simulink model "quad2_jump"  (R2015b)
settings: Solver=FixedStepAuto  StartTime=0.0  StopTime=10  FixedStep=1e-4  MinStep=1e-4  RelTol=1e-2  AbsTol=1e-6
InitFcn:
  | init_quad;
StartFcn:
  | init_quad;
undefined symbols (not defined in the file or in its folder): body, ctrl, planner, sigbuilder_block, X, Y, Z
libraries: nesl_utility x61, sm_lib x41, simulink x4, Contact_Forces_Lib x4, Parts_Lib x4
(part 3 of 3)

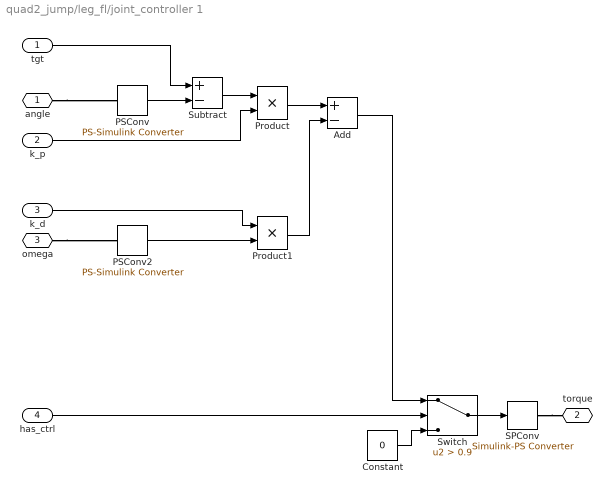
== system quad2_jump/leg_fl/joint_controller 1 ==
  tgt : Inport
  k_p : Inport  Port=2
  k_d : Inport  Port=3
  has_ctrl : Inport  Port=4
  Add : Sum  Inputs=+-
  Constant : Constant  Value=0
  PSConv : nesl_utility/PS-Simulink Converter  PhysicalDomain=network_engine_domain  SubClassName=ps_output  LeftPortType=input  RightPortType=output  PseudoPeriodic=off  Frequencies=[]  Unit=1  AffineConversion=off
  PSConv2 : nesl_utility/PS-Simulink Converter  PhysicalDomain=network_engine_domain  SubClassName=ps_output  LeftPortType=input  RightPortType=output  PseudoPeriodic=off  Frequencies=[]  Unit=1  AffineConversion=off
  Product : Product  Inputs=**
  Product1 : Product  Inputs=**
  SPConv : nesl_utility/Simulink-PS Converter  PhysicalDomain=network_engine_domain  SubClassName=ps_input  LeftPortType=input  RightPortType=output  PseudoPeriodic=off  Frequencies=[]  NoiseDistribution=none  NoiseParameters=[]  Unit=1  AffineConversion=off  InputFiltering=on  SimscapeFilterOrder=2  InputFilterTimeConstant=0.001  UdotUserProvided=1
  Subtract : Sum  Inputs=+-
  Switch : Switch  Criteria=u2 > Threshold  Threshold=0.9
  angle : PMIOPort  Port=1  Side=Left
  torque : PMIOPort  Port=2  Side=Right
  omega : PMIOPort  Port=3  Side=Left
  wires:
  Product1/1 -> Add/2
  tgt/1 -> Subtract/1
  Product/1 -> Add/1
  PSConv/1 -> Subtract/2
  Subtract/1 -> Product/1
  k_d/1 -> Product1/1
  PSConv2/1 -> Product1/2
  k_p/1 -> Product/2
  Switch/1 -> SPConv/1
  has_ctrl/1 -> Switch/2
  Constant/1 -> Switch/3
  Add/1 -> Switch/1
  connections:
  angle/RConn1 -- PSConv/LConn1
  omega/RConn1 -- PSConv2/LConn1
  SPConv/RConn1 -- torque/RConn1

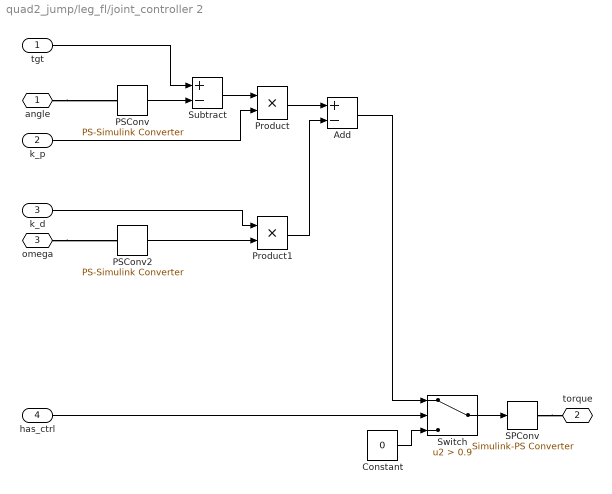
== system quad2_jump/leg_fl/joint_controller 2 ==
  tgt : Inport
  k_p : Inport  Port=2
  k_d : Inport  Port=3
  has_ctrl : Inport  Port=4
  Add : Sum  Inputs=+-
  Constant : Constant  Value=0
  PSConv : nesl_utility/PS-Simulink Converter  PhysicalDomain=network_engine_domain  SubClassName=ps_output  LeftPortType=input  RightPortType=output  PseudoPeriodic=off  Frequencies=[]  Unit=1  AffineConversion=off
  PSConv2 : nesl_utility/PS-Simulink Converter  PhysicalDomain=network_engine_domain  SubClassName=ps_output  LeftPortType=input  RightPortType=output  PseudoPeriodic=off  Frequencies=[]  Unit=1  AffineConversion=off
  Product : Product  Inputs=**
  Product1 : Product  Inputs=**
  SPConv : nesl_utility/Simulink-PS Converter  PhysicalDomain=network_engine_domain  SubClassName=ps_input  LeftPortType=input  RightPortType=output  PseudoPeriodic=off  Frequencies=[]  NoiseDistribution=none  NoiseParameters=[]  Unit=1  AffineConversion=off  InputFiltering=on  SimscapeFilterOrder=2  InputFilterTimeConstant=0.001  UdotUserProvided=1
  Subtract : Sum  Inputs=+-
  Switch : Switch  Criteria=u2 > Threshold  Threshold=0.9
  angle : PMIOPort  Port=1  Side=Left
  torque : PMIOPort  Port=2  Side=Right
  omega : PMIOPort  Port=3  Side=Left
  wires:
  Product1/1 -> Add/2
  tgt/1 -> Subtract/1
  Product/1 -> Add/1
  PSConv/1 -> Subtract/2
  Subtract/1 -> Product/1
  k_d/1 -> Product1/1
  PSConv2/1 -> Product1/2
  k_p/1 -> Product/2
  Switch/1 -> SPConv/1
  has_ctrl/1 -> Switch/2
  Constant/1 -> Switch/3
  Add/1 -> Switch/1
  connections:
  angle/RConn1 -- PSConv/LConn1
  omega/RConn1 -- PSConv2/LConn1
  SPConv/RConn1 -- torque/RConn1

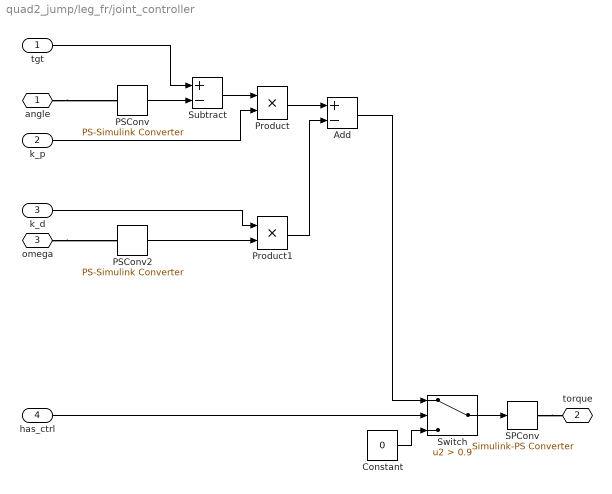
== system quad2_jump/leg_fr/joint_controller  ==
  tgt : Inport
  k_p : Inport  Port=2
  k_d : Inport  Port=3
  has_ctrl : Inport  Port=4
  Add : Sum  Inputs=+-
  Constant : Constant  Value=0
  PSConv : nesl_utility/PS-Simulink Converter  PhysicalDomain=network_engine_domain  SubClassName=ps_output  LeftPortType=input  RightPortType=output  PseudoPeriodic=off  Frequencies=[]  Unit=1  AffineConversion=off
  PSConv2 : nesl_utility/PS-Simulink Converter  PhysicalDomain=network_engine_domain  SubClassName=ps_output  LeftPortType=input  RightPortType=output  PseudoPeriodic=off  Frequencies=[]  Unit=1  AffineConversion=off
  Product : Product  Inputs=**
  Product1 : Product  Inputs=**
  SPConv : nesl_utility/Simulink-PS Converter  PhysicalDomain=network_engine_domain  SubClassName=ps_input  LeftPortType=input  RightPortType=output  PseudoPeriodic=off  Frequencies=[]  NoiseDistribution=none  NoiseParameters=[]  Unit=1  AffineConversion=off  InputFiltering=on  SimscapeFilterOrder=2  InputFilterTimeConstant=0.001  UdotUserProvided=1
  Subtract : Sum  Inputs=+-
  Switch : Switch  Criteria=u2 > Threshold  Threshold=0.9
  angle : PMIOPort  Port=1  Side=Left
  torque : PMIOPort  Port=2  Side=Right
  omega : PMIOPort  Port=3  Side=Left
  wires:
  Product1/1 -> Add/2
  tgt/1 -> Subtract/1
  Product/1 -> Add/1
  PSConv/1 -> Subtract/2
  Subtract/1 -> Product/1
  k_d/1 -> Product1/1
  PSConv2/1 -> Product1/2
  k_p/1 -> Product/2
  Switch/1 -> SPConv/1
  has_ctrl/1 -> Switch/2
  Constant/1 -> Switch/3
  Add/1 -> Switch/1
  connections:
  angle/RConn1 -- PSConv/LConn1
  omega/RConn1 -- PSConv2/LConn1
  SPConv/RConn1 -- torque/RConn1

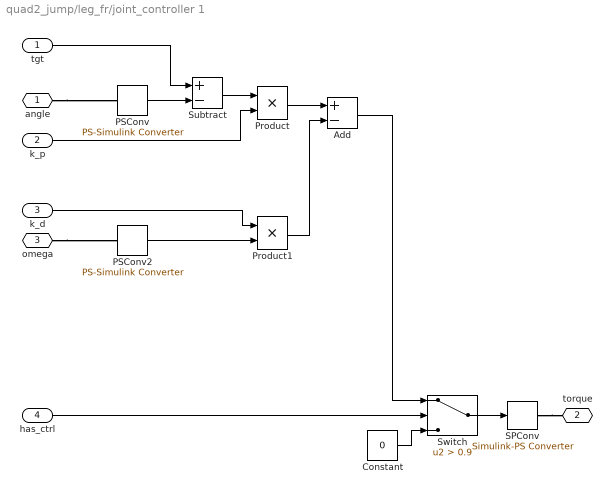
== system quad2_jump/leg_fr/joint_controller 1 ==
  tgt : Inport
  k_p : Inport  Port=2
  k_d : Inport  Port=3
  has_ctrl : Inport  Port=4
  Add : Sum  Inputs=+-
  Constant : Constant  Value=0
  PSConv : nesl_utility/PS-Simulink Converter  PhysicalDomain=network_engine_domain  SubClassName=ps_output  LeftPortType=input  RightPortType=output  PseudoPeriodic=off  Frequencies=[]  Unit=1  AffineConversion=off
  PSConv2 : nesl_utility/PS-Simulink Converter  PhysicalDomain=network_engine_domain  SubClassName=ps_output  LeftPortType=input  RightPortType=output  PseudoPeriodic=off  Frequencies=[]  Unit=1  AffineConversion=off
  Product : Product  Inputs=**
  Product1 : Product  Inputs=**
  SPConv : nesl_utility/Simulink-PS Converter  PhysicalDomain=network_engine_domain  SubClassName=ps_input  LeftPortType=input  RightPortType=output  PseudoPeriodic=off  Frequencies=[]  NoiseDistribution=none  NoiseParameters=[]  Unit=1  AffineConversion=off  InputFiltering=on  SimscapeFilterOrder=2  InputFilterTimeConstant=0.001  UdotUserProvided=1
  Subtract : Sum  Inputs=+-
  Switch : Switch  Criteria=u2 > Threshold  Threshold=0.9
  angle : PMIOPort  Port=1  Side=Left
  torque : PMIOPort  Port=2  Side=Right
  omega : PMIOPort  Port=3  Side=Left
  wires:
  Product1/1 -> Add/2
  tgt/1 -> Subtract/1
  Product/1 -> Add/1
  PSConv/1 -> Subtract/2
  Subtract/1 -> Product/1
  k_d/1 -> Product1/1
  PSConv2/1 -> Product1/2
  k_p/1 -> Product/2
  Switch/1 -> SPConv/1
  has_ctrl/1 -> Switch/2
  Constant/1 -> Switch/3
  Add/1 -> Switch/1
  connections:
  angle/RConn1 -- PSConv/LConn1
  omega/RConn1 -- PSConv2/LConn1
  SPConv/RConn1 -- torque/RConn1

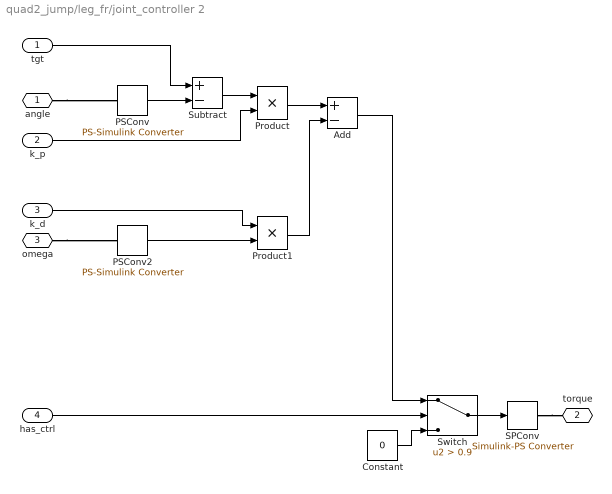
== system quad2_jump/leg_fr/joint_controller 2 ==
  tgt : Inport
  k_p : Inport  Port=2
  k_d : Inport  Port=3
  has_ctrl : Inport  Port=4
  Add : Sum  Inputs=+-
  Constant : Constant  Value=0
  PSConv : nesl_utility/PS-Simulink Converter  PhysicalDomain=network_engine_domain  SubClassName=ps_output  LeftPortType=input  RightPortType=output  PseudoPeriodic=off  Frequencies=[]  Unit=1  AffineConversion=off
  PSConv2 : nesl_utility/PS-Simulink Converter  PhysicalDomain=network_engine_domain  SubClassName=ps_output  LeftPortType=input  RightPortType=output  PseudoPeriodic=off  Frequencies=[]  Unit=1  AffineConversion=off
  Product : Product  Inputs=**
  Product1 : Product  Inputs=**
  SPConv : nesl_utility/Simulink-PS Converter  PhysicalDomain=network_engine_domain  SubClassName=ps_input  LeftPortType=input  RightPortType=output  PseudoPeriodic=off  Frequencies=[]  NoiseDistribution=none  NoiseParameters=[]  Unit=1  AffineConversion=off  InputFiltering=on  SimscapeFilterOrder=2  InputFilterTimeConstant=0.001  UdotUserProvided=1
  Subtract : Sum  Inputs=+-
  Switch : Switch  Criteria=u2 > Threshold  Threshold=0.9
  angle : PMIOPort  Port=1  Side=Left
  torque : PMIOPort  Port=2  Side=Right
  omega : PMIOPort  Port=3  Side=Left
  wires:
  Product1/1 -> Add/2
  tgt/1 -> Subtract/1
  Product/1 -> Add/1
  PSConv/1 -> Subtract/2
  Subtract/1 -> Product/1
  k_d/1 -> Product1/1
  PSConv2/1 -> Product1/2
  k_p/1 -> Product/2
  Switch/1 -> SPConv/1
  has_ctrl/1 -> Switch/2
  Constant/1 -> Switch/3
  Add/1 -> Switch/1
  connections:
  angle/RConn1 -- PSConv/LConn1
  omega/RConn1 -- PSConv2/LConn1
  SPConv/RConn1 -- torque/RConn1

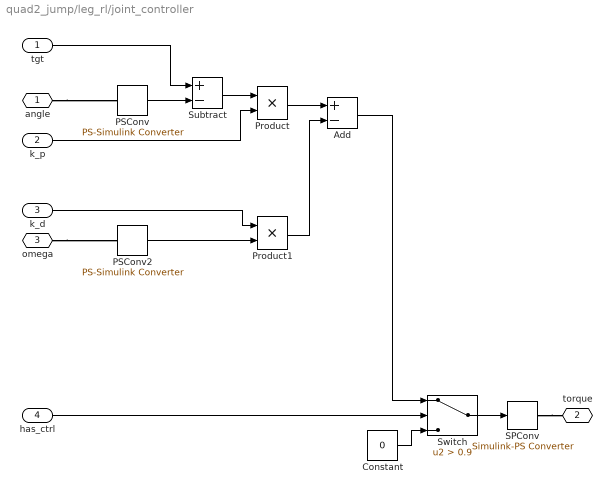
== system quad2_jump/leg_rl/joint_controller  ==
  tgt : Inport
  k_p : Inport  Port=2
  k_d : Inport  Port=3
  has_ctrl : Inport  Port=4
  Add : Sum  Inputs=+-
  Constant : Constant  Value=0
  PSConv : nesl_utility/PS-Simulink Converter  PhysicalDomain=network_engine_domain  SubClassName=ps_output  LeftPortType=input  RightPortType=output  PseudoPeriodic=off  Frequencies=[]  Unit=1  AffineConversion=off
  PSConv2 : nesl_utility/PS-Simulink Converter  PhysicalDomain=network_engine_domain  SubClassName=ps_output  LeftPortType=input  RightPortType=output  PseudoPeriodic=off  Frequencies=[]  Unit=1  AffineConversion=off
  Product : Product  Inputs=**
  Product1 : Product  Inputs=**
  SPConv : nesl_utility/Simulink-PS Converter  PhysicalDomain=network_engine_domain  SubClassName=ps_input  LeftPortType=input  RightPortType=output  PseudoPeriodic=off  Frequencies=[]  NoiseDistribution=none  NoiseParameters=[]  Unit=1  AffineConversion=off  InputFiltering=on  SimscapeFilterOrder=2  InputFilterTimeConstant=0.001  UdotUserProvided=1
  Subtract : Sum  Inputs=+-
  Switch : Switch  Criteria=u2 > Threshold  Threshold=0.9
  angle : PMIOPort  Port=1  Side=Left
  torque : PMIOPort  Port=2  Side=Right
  omega : PMIOPort  Port=3  Side=Left
  wires:
  Product1/1 -> Add/2
  tgt/1 -> Subtract/1
  Product/1 -> Add/1
  PSConv/1 -> Subtract/2
  Subtract/1 -> Product/1
  k_d/1 -> Product1/1
  PSConv2/1 -> Product1/2
  k_p/1 -> Product/2
  Switch/1 -> SPConv/1
  has_ctrl/1 -> Switch/2
  Constant/1 -> Switch/3
  Add/1 -> Switch/1
  connections:
  angle/RConn1 -- PSConv/LConn1
  omega/RConn1 -- PSConv2/LConn1
  SPConv/RConn1 -- torque/RConn1

== system quad2_jump/leg_rl/joint_controller 1 ==
  tgt : Inport
  k_p : Inport  Port=2
  k_d : Inport  Port=3
  has_ctrl : Inport  Port=4
  Add : Sum  Inputs=+-
  Constant : Constant  Value=0
  PSConv : nesl_utility/PS-Simulink Converter  PhysicalDomain=network_engine_domain  SubClassName=ps_output  LeftPortType=input  RightPortType=output  PseudoPeriodic=off  Frequencies=[]  Unit=1  AffineConversion=off
  PSConv2 : nesl_utility/PS-Simulink Converter  PhysicalDomain=network_engine_domain  SubClassName=ps_output  LeftPortType=input  RightPortType=output  PseudoPeriodic=off  Frequencies=[]  Unit=1  AffineConversion=off
  Product : Product  Inputs=**
  Product1 : Product  Inputs=**
  SPConv : nesl_utility/Simulink-PS Converter  PhysicalDomain=network_engine_domain  SubClassName=ps_input  LeftPortType=input  RightPortType=output  PseudoPeriodic=off  Frequencies=[]  NoiseDistribution=none  NoiseParameters=[]  Unit=1  AffineConversion=off  InputFiltering=on  SimscapeFilterOrder=2  InputFilterTimeConstant=0.001  UdotUserProvided=1
  Subtract : Sum  Inputs=+-
  Switch : Switch  Criteria=u2 > Threshold  Threshold=0.9
  angle : PMIOPort  Port=1  Side=Left
  torque : PMIOPort  Port=2  Side=Right
  omega : PMIOPort  Port=3  Side=Left
  wires:
  Product1/1 -> Add/2
  tgt/1 -> Subtract/1
  Product/1 -> Add/1
  PSConv/1 -> Subtract/2
  Subtract/1 -> Product/1
  k_d/1 -> Product1/1
  PSConv2/1 -> Product1/2
  k_p/1 -> Product/2
  Switch/1 -> SPConv/1
  has_ctrl/1 -> Switch/2
  Constant/1 -> Switch/3
  Add/1 -> Switch/1
  connections:
  angle/RConn1 -- PSConv/LConn1
  omega/RConn1 -- PSConv2/LConn1
  SPConv/RConn1 -- torque/RConn1

== system quad2_jump/leg_rl/joint_controller 2 ==
  tgt : Inport
  k_p : Inport  Port=2
  k_d : Inport  Port=3
  has_ctrl : Inport  Port=4
  Add : Sum  Inputs=+-
  Constant : Constant  Value=0
  PSConv : nesl_utility/PS-Simulink Converter  PhysicalDomain=network_engine_domain  SubClassName=ps_output  LeftPortType=input  RightPortType=output  PseudoPeriodic=off  Frequencies=[]  Unit=1  AffineConversion=off
  PSConv2 : nesl_utility/PS-Simulink Converter  PhysicalDomain=network_engine_domain  SubClassName=ps_output  LeftPortType=input  RightPortType=output  PseudoPeriodic=off  Frequencies=[]  Unit=1  AffineConversion=off
  Product : Product  Inputs=**
  Product1 : Product  Inputs=**
  SPConv : nesl_utility/Simulink-PS Converter  PhysicalDomain=network_engine_domain  SubClassName=ps_input  LeftPortType=input  RightPortType=output  PseudoPeriodic=off  Frequencies=[]  NoiseDistribution=none  NoiseParameters=[]  Unit=1  AffineConversion=off  InputFiltering=on  SimscapeFilterOrder=2  InputFilterTimeConstant=0.001  UdotUserProvided=1
  Subtract : Sum  Inputs=+-
  Switch : Switch  Criteria=u2 > Threshold  Threshold=0.9
  angle : PMIOPort  Port=1  Side=Left
  torque : PMIOPort  Port=2  Side=Right
  omega : PMIOPort  Port=3  Side=Left
  wires:
  Product1/1 -> Add/2
  tgt/1 -> Subtract/1
  Product/1 -> Add/1
  PSConv/1 -> Subtract/2
  Subtract/1 -> Product/1
  k_d/1 -> Product1/1
  PSConv2/1 -> Product1/2
  k_p/1 -> Product/2
  Switch/1 -> SPConv/1
  has_ctrl/1 -> Switch/2
  Constant/1 -> Switch/3
  Add/1 -> Switch/1
  connections:
  angle/RConn1 -- PSConv/LConn1
  omega/RConn1 -- PSConv2/LConn1
  SPConv/RConn1 -- torque/RConn1

== system quad2_jump/leg_rr/joint_controller  ==
  tgt : Inport
  k_p : Inport  Port=2
  k_d : Inport  Port=3
  has_ctrl : Inport  Port=4
  Add : Sum  Inputs=+-
  Constant : Constant  Value=0
  PSConv : nesl_utility/PS-Simulink Converter  PhysicalDomain=network_engine_domain  SubClassName=ps_output  LeftPortType=input  RightPortType=output  PseudoPeriodic=off  Frequencies=[]  Unit=1  AffineConversion=off
  PSConv2 : nesl_utility/PS-Simulink Converter  PhysicalDomain=network_engine_domain  SubClassName=ps_output  LeftPortType=input  RightPortType=output  PseudoPeriodic=off  Frequencies=[]  Unit=1  AffineConversion=off
  Product : Product  Inputs=**
  Product1 : Product  Inputs=**
  SPConv : nesl_utility/Simulink-PS Converter  PhysicalDomain=network_engine_domain  SubClassName=ps_input  LeftPortType=input  RightPortType=output  PseudoPeriodic=off  Frequencies=[]  NoiseDistribution=none  NoiseParameters=[]  Unit=1  AffineConversion=off  InputFiltering=on  SimscapeFilterOrder=2  InputFilterTimeConstant=0.001  UdotUserProvided=1
  Subtract : Sum  Inputs=+-
  Switch : Switch  Criteria=u2 > Threshold  Threshold=0.9
  angle : PMIOPort  Port=1  Side=Left
  torque : PMIOPort  Port=2  Side=Right
  omega : PMIOPort  Port=3  Side=Left
  wires:
  Product1/1 -> Add/2
  tgt/1 -> Subtract/1
  Product/1 -> Add/1
  PSConv/1 -> Subtract/2
  Subtract/1 -> Product/1
  k_d/1 -> Product1/1
  PSConv2/1 -> Product1/2
  k_p/1 -> Product/2
  Switch/1 -> SPConv/1
  has_ctrl/1 -> Switch/2
  Constant/1 -> Switch/3
  Add/1 -> Switch/1
  connections:
  angle/RConn1 -- PSConv/LConn1
  omega/RConn1 -- PSConv2/LConn1
  SPConv/RConn1 -- torque/RConn1

== system quad2_jump/leg_rr/joint_controller 1 ==
  tgt : Inport
  k_p : Inport  Port=2
  k_d : Inport  Port=3
  has_ctrl : Inport  Port=4
  Add : Sum  Inputs=+-
  Constant : Constant  Value=0
  PSConv : nesl_utility/PS-Simulink Converter  PhysicalDomain=network_engine_domain  SubClassName=ps_output  LeftPortType=input  RightPortType=output  PseudoPeriodic=off  Frequencies=[]  Unit=1  AffineConversion=off
  PSConv2 : nesl_utility/PS-Simulink Converter  PhysicalDomain=network_engine_domain  SubClassName=ps_output  LeftPortType=input  RightPortType=output  PseudoPeriodic=off  Frequencies=[]  Unit=1  AffineConversion=off
  Product : Product  Inputs=**
  Product1 : Product  Inputs=**
  SPConv : nesl_utility/Simulink-PS Converter  PhysicalDomain=network_engine_domain  SubClassName=ps_input  LeftPortType=input  RightPortType=output  PseudoPeriodic=off  Frequencies=[]  NoiseDistribution=none  NoiseParameters=[]  Unit=1  AffineConversion=off  InputFiltering=on  SimscapeFilterOrder=2  InputFilterTimeConstant=0.001  UdotUserProvided=1
  Subtract : Sum  Inputs=+-
  Switch : Switch  Criteria=u2 > Threshold  Threshold=0.9
  angle : PMIOPort  Port=1  Side=Left
  torque : PMIOPort  Port=2  Side=Right
  omega : PMIOPort  Port=3  Side=Left
  wires:
  Product1/1 -> Add/2
  tgt/1 -> Subtract/1
  Product/1 -> Add/1
  PSConv/1 -> Subtract/2
  Subtract/1 -> Product/1
  k_d/1 -> Product1/1
  PSConv2/1 -> Product1/2
  k_p/1 -> Product/2
  Switch/1 -> SPConv/1
  has_ctrl/1 -> Switch/2
  Constant/1 -> Switch/3
  Add/1 -> Switch/1
  connections:
  angle/RConn1 -- PSConv/LConn1
  omega/RConn1 -- PSConv2/LConn1
  SPConv/RConn1 -- torque/RConn1

== system quad2_jump/leg_rr/joint_controller 2 ==
  tgt : Inport
  k_p : Inport  Port=2
  k_d : Inport  Port=3
  has_ctrl : Inport  Port=4
  Add : Sum  Inputs=+-
  Constant : Constant  Value=0
  PSConv : nesl_utility/PS-Simulink Converter  PhysicalDomain=network_engine_domain  SubClassName=ps_output  LeftPortType=input  RightPortType=output  PseudoPeriodic=off  Frequencies=[]  Unit=1  AffineConversion=off
  PSConv2 : nesl_utility/PS-Simulink Converter  PhysicalDomain=network_engine_domain  SubClassName=ps_output  LeftPortType=input  RightPortType=output  PseudoPeriodic=off  Frequencies=[]  Unit=1  AffineConversion=off
  Product : Product  Inputs=**
  Product1 : Product  Inputs=**
  SPConv : nesl_utility/Simulink-PS Converter  PhysicalDomain=network_engine_domain  SubClassName=ps_input  LeftPortType=input  RightPortType=output  PseudoPeriodic=off  Frequencies=[]  NoiseDistribution=none  NoiseParameters=[]  Unit=1  AffineConversion=off  InputFiltering=on  SimscapeFilterOrder=2  InputFilterTimeConstant=0.001  UdotUserProvided=1
  Subtract : Sum  Inputs=+-
  Switch : Switch  Criteria=u2 > Threshold  Threshold=0.9
  angle : PMIOPort  Port=1  Side=Left
  torque : PMIOPort  Port=2  Side=Right
  omega : PMIOPort  Port=3  Side=Left
  wires:
  Product1/1 -> Add/2
  tgt/1 -> Subtract/1
  Product/1 -> Add/1
  PSConv/1 -> Subtract/2
  Subtract/1 -> Product/1
  k_d/1 -> Product1/1
  PSConv2/1 -> Product1/2
  k_p/1 -> Product/2
  Switch/1 -> SPConv/1
  has_ctrl/1 -> Switch/2
  Constant/1 -> Switch/3
  Add/1 -> Switch/1
  connections:
  angle/RConn1 -- PSConv/LConn1
  omega/RConn1 -- PSConv2/LConn1
  SPConv/RConn1 -- torque/RConn1

== matlab function quad2_jump/Controller ==
  data: fl_ang_s input; fl_tgt_ang_s output; fl_ang_u input; fl_ang_k input; fr_ang_s input; fr_ang_u input; fr_ang_k input; rl_ang_s input; rl_ang_u input; rl_ang_k input; rr_ang_s input; rr_ang_u input; rr_ang_k input; in_tgt_body_theta input; body_R input; body_z input; body_vx input; contact_state input; fl_tgt_ang_u output; fl_has_ctrl_u output; fl_tgt_ang_k output; fr_tgt_ang_s output; fr_tgt_ang_u output; fr_has_ctrl_u output; fr_tgt_ang_k output; rl_tgt_ang_s output; rl_tgt_ang_u output; rl_has_ctrl_u output; rl_tgt_ang_k output; rr_tgt_ang_s output; rr_tgt_ang_u output; rr_has_ctrl_u output; rr_tgt_ang_k output; body parameter; planner parameter; ctrl_state output
function [fl_tgt_ang_s, fl_tgt_ang_u, fl_has_ctrl_u, fl_tgt_ang_k,...
    fr_tgt_ang_s, fr_tgt_ang_u, fr_has_ctrl_u, fr_tgt_ang_k,...
    rl_tgt_ang_s, rl_tgt_ang_u, rl_has_ctrl_u, rl_tgt_ang_k,...
    rr_tgt_ang_s, rr_tgt_ang_u, rr_has_ctrl_u, rr_tgt_ang_k, ctrl_state]...
      = fcn(fl_ang_s, fl_ang_u, fl_ang_k, ...
                  fr_ang_s, fr_ang_u, fr_ang_k, ...
                  rl_ang_s, rl_ang_u, rl_ang_k, ...
                  rr_ang_s, rr_ang_u, rr_ang_k, ...
                  in_tgt_body_theta, body_R, body_z, body_vx,  contact_state, body, planner)
              
              
% forward kinematics
fl_end_effector = forward_kinematics(fl_ang_s, fl_ang_u, fl_ang_k, body); 
rl_end_effector = forward_kinematics(rl_ang_s, rl_ang_u, rl_ang_k, body);
fr_end_effector = forward_kinematics(fr_ang_s, fr_ang_u, fr_ang_k, body);
rr_end_effector = forward_kinematics(rr_ang_s, rr_ang_u, rr_ang_k, body); 

% distance from center of mass to shoulder
fl_offset = [body.shoulder_distance;body.y_length/2+body.shoulder_size/2;0];
fr_offset = [body.shoulder_distance;-body.y_length/2-body.shoulder_size/2;0];
rl_offset = [-body.shoulder_distance;body.y_length/2+body.shoulder_size/2;0];
rr_offset = [-body.shoulder_distance;-body.y_length/2-body.shoulder_size/2;0];

%virtual leg1
virtual_leg1 = (fl_end_effector + fl_offset + rr_end_effector + rr_offset)*0.5;
%virtual leg2
virtual_leg2 = (fr_end_effector + fr_offset + rl_end_effector + rl_offset)*0.5;
         
%decide state 
persistent state;
persistent timer;
persistent timer2;
persistent record_helper;
if isempty(state)
    state = 0;
end
if isempty(timer)
    timer = 0;
end
if isempty(timer2)
    timer2 = 0;
end
if isempty(record_helper)
    record_helper = 0;
end


% init variables
tgt_body_theta = 0;
tgt_virtual_leg1 = [0;0;-planner.stand_height+planner.touch_down_height];
tgt_virtual_leg2 = [0;0;-planner.stand_height+planner.touch_down_height];
no_u_ctrl = [0 0 0 0];
if state == 0
    tgt_body_theta = 0;
    % set target virtual legs according to state
    tgt_virtual_leg1 = [0;0;-planner.stand_height+planner.touch_down_height];
    tgt_virtual_leg2 = [0;0;-planner.stand_height+planner.touch_down_height];
    
    if contact_state(1) == 1 && contact_state(2) == 1 && contact_state(3) == 1 && contact_state(4) == 1
        %all foot on ground
        if body_vx < 0.1 
            timer = timer + 1;
        else
            timer = 0;
        end
        if timer > 1500
            state = 1;
            timer = 0;
        end
    end
elseif state == 1
    tgt_body_theta = 0;
    tgt_virtual_leg1 = [0;0;-planner.stand_height+planner.touch_down_height];
    tgt_virtual_leg2 = [0;0;-planner.stand_height+planner.touch_down_height];
%     move_theta = 2*pi/180;
%     move_leg_R = [cos(move_theta) 0 sin(move_theta);
%         0 1 0;
%         -sin(move_theta) 0 cos(move_theta)];
%     tgt_virtual_leg1 = move_leg_R*tgt_virtual_leg1;
%     tgt_virtual_leg2 = move_leg_R*tgt_virtual_leg2;
    if body_vx < 0.1
        timer = timer + 1;
    else
        timer = 0;
    end
    if timer > 42000
        state = 2;
        timer = 0;
        timer2 = 0;
        record_helper = 1.0;
    end
elseif state == 2 % start to move forward
    tgt_body_theta = 0;
    if contact_state(1) == 1 && contact_state(2) == 1 && contact_state(3) == 1 && contact_state(4) == 1
        %length_coef = 1.0 - timer2/8600*0.5;
        move_theta = timer2/4000*20/180*pi;
        timer2 = timer2 + 2;
    else
%         length_coef = record_helper;
        move_theta = 0;
    end
    tgt_virtual_leg1 = [0;0;-planner.stand_height+planner.touch_down_height];
    tgt_virtual_leg2 = [0;0;-planner.stand_height+planner.touch_down_height];
 
%     move_theta = timer2/1000*3/180*pi;
    move_leg_R = [cos(move_theta) 0 sin(move_theta);
        0 1 0;
        -sin(move_theta) 0 cos(move_theta)];    
    tgt_virtual_leg1 = move_leg_R*tgt_virtual_leg1;
    tgt_virtual_leg2 = move_leg_R*tgt_virtual_leg2;
%     timer2 = timer2 + 1;
    if contact_state(1) == 1 && contact_state(2) == 1 && contact_state(3) == 1 && contact_state(4) == 1 && body_vx > 0.4
        timer = timer + 1;
    else
        timer = 0;
    end
%     record_helper = length_coef;
%     if contact_state(1) == 1 && contact_state(2) == 1 && contact_state(3) == 1 && contact_state(4) == 1 && length_coef <= 0.68
    if timer > 200
        state = 3;
        timer = 0;
        timer2 = 0;
%         record_helper = length_coef;
    end
    if timer2 > 9000
        timer2 = 9000;
    end
elseif state == 3 % virtual leg 1 moves
    tgt_body_theta = in_tgt_body_theta;
    tgt_virtual_leg1 = [0;0;-planner.stand_height+planner.touch_down_height];
    tgt_virtual_leg2 = [0;0;-planner.stand_height+planner.touch_down_height];
%  
    move_theta = 10/180*pi;
    move_leg_R = [cos(move_theta) 0 sin(move_theta);
        0 1 0;
        -sin(move_theta) 0 cos(move_theta)];    
    length_coef = 0.8+ timer2/9000*0.2;
    tgt_virtual_leg1 = move_leg_R*length_coef*tgt_virtual_leg1;
%     tgt_virtual_leg2 = move_leg_R*tgt_virtual_leg2;
    no_u_ctrl = [0 1 1 0];
%     tgt_virtual_leg1 = [0;0;-planner.flight_height+planner.touch_down_height];
%     tgt_virtual_leg2 = virtual_leg2;
%     length_coef = record_helper + timer2/8600*0.5;
%     if length_coef > 1.2
%         length_coef = 1.2;
%     end
%     tgt_virtual_leg1 = length_coef*[0;0;-planner.stand_height+planner.touch_down_height];
%     tgt_virtual_leg2 = length_coef*[0;0;-planner.stand_height+planner.touch_down_height];
%     
	timer2 = timer2 + 2;
    if timer2 > 9000
        timer2 = 9000;
    end
    if contact_state(1) == 1 && contact_state(4) == 1 && length_coef >0.99
        timer = timer + 1;
    end
    if timer > 200
        state = 4;
        timer = 0;
        timer2 = 0;
    end
elseif state == 4
    tgt_body_theta = in_tgt_body_theta;
    tgt_virtual_leg1 = [0;0;-planner.stand_height+planner.touch_down_height];
    tgt_virtual_leg2 = [0;0;-planner.stand_height+planner.touch_down_height];
%  
    move_theta = 10/180*pi;
    move_leg_R = [cos(move_theta) 0 sin(move_theta);
        0 1 0;
        -sin(move_theta) 0 cos(move_theta)];    
    length_coef = 0.8+ timer2/9000*0.2;
    tgt_virtual_leg2 = move_leg_R*length_coef*tgt_virtual_leg2;
    no_u_ctrl = [1 0 0 1];
    	timer2 = timer2 + 2;
    if timer2 > 9000
        timer2 = 9000;
    end
    if contact_state(2) == 1 && contact_state(3) == 1 && length_coef >0.99
        timer = timer + 1;
    end
    if timer > 200
        state = 3;
        timer = 0;
        timer2 = 0;
    end
end
ctrl_state = state;

% confine range of tgt_virtual legs

% track tgt body angle
tgt_body_R = [cos(tgt_body_theta) 0 sin(tgt_body_theta);0 1 0;-sin(tgt_body_theta) 0 cos(tgt_body_theta)];

tgt_virtual_leg1_b = tgt_body_R'*tgt_virtual_leg1;
tgt_virtual_leg2_b = tgt_body_R'*tgt_virtual_leg2;
% TODO: need to change if two legs move together once 
if contact_state(1) == 0 && contact_state(4) == 0
    tgt_fl_end_effector = tgt_virtual_leg1_b+body_R'*fl_offset;
    tgt_rr_end_effector = tgt_virtual_leg1_b+body_R'*rr_offset;
else
    tgt_fl_end_effector = tgt_virtual_leg1_b+tgt_body_R'*fl_offset;
    tgt_rr_end_effector = tgt_virtual_leg1_b+tgt_body_R'*rr_offset;
end
if contact_state(2) == 0 && contact_state(3) == 0 
    tgt_fr_end_effector = tgt_virtual_leg2_b+body_R'*fr_offset;
    tgt_rl_end_effector = tgt_virtual_leg2_b+body_R'*rl_offset;
else
    tgt_fr_end_effector = tgt_virtual_leg2_b+tgt_body_R'*fr_offset;
    tgt_rl_end_effector = tgt_virtual_leg2_b+tgt_body_R'*rl_offset;
end

move_fl_end_effector = tgt_fl_end_effector-fl_offset;
move_fr_end_effector = tgt_fr_end_effector-fr_offset;
move_rl_end_effector = tgt_rl_end_effector-rl_offset;
move_rr_end_effector = tgt_rr_end_effector-rr_offset;


% move_fl_end_effector = fl_end_effector + 0.8* (tgt_fl_end_effector-fl_offset -fl_end_effector);
% move_fr_end_effector = fr_end_effector + 0.8* (tgt_fr_end_effector-fr_offset -fr_end_effector);
% move_rl_end_effector = rl_end_effector + 0.8* (tgt_rl_end_effector-rl_offset -rl_end_effector);
% move_rr_end_effector = rr_end_effector + 0.8* (tgt_rr_end_effector-rr_offset -rr_end_effector);
% from target virtual legs to joint angles (inverse kinematics)
[inv_s,inv_u,inv_k] = inverse_kinematics(move_fl_end_effector, body);

fl_tgt_ang_s = inv_s; % x-axis, theta
fl_tgt_ang_u = inv_u;         % y-axis, theta
if no_u_ctrl(1) == 1
    fl_has_ctrl_u = 0;
else
    fl_has_ctrl_u = 1;
end
fl_tgt_ang_k = inv_k; % y-axis, theta

[inv_s,inv_u,inv_k] = inverse_kinematics(move_fr_end_effector, body);
fr_tgt_ang_s = inv_s;
fr_tgt_ang_u = inv_u;
if no_u_ctrl(2) == 1
    fr_has_ctrl_u = 0;
else
    fr_has_ctrl_u = 1;
end
fr_tgt_ang_k = inv_k;

[inv_s,inv_u,inv_k] = inverse_kinematics(move_rl_end_effector, body);
rl_tgt_ang_s = inv_s;
rl_tgt_ang_u = inv_u;
if no_u_ctrl(3) == 1
    rl_has_ctrl_u = 0;
else
    rl_has_ctrl_u = 1;
end
rl_tgt_ang_k = inv_k;

[inv_s,inv_u,inv_k] = inverse_kinematics(move_rr_end_effector, body);
rr_tgt_ang_s = inv_s;
rr_tgt_ang_u = inv_u;
if no_u_ctrl(4) == 1
    rr_has_ctrl_u = 0;
else
    rr_has_ctrl_u = 1;
end
rr_tgt_ang_k = inv_k;  

% dummy output just for testing              
% fl_tgt_ang_s = 0*pi/180; % x-axis, theta
% fl_tgt_ang_u = 30*pi/180;         % y-axis, theta
% fl_has_ctrl_u = 1;
% fl_tgt_ang_k = -60*pi/180; % y-axis, theta
% 
% fr_tgt_ang_s = 0*pi/180;
% fr_tgt_ang_u = 30*pi/180;
% fr_has_ctrl_u = 1;
% fr_tgt_ang_k = -60*pi/180;
% 
% rl_tgt_ang_s = 0*pi/180;
% rl_tgt_ang_u = 30*pi/180;
% rl_has_ctrl_u = 1;
% rl_tgt_ang_k = -60*pi/180;
% 
% rr_tgt_ang_s = 0*pi/180;
% rr_tgt_ang_u = 30*pi/180;
% rr_has_ctrl_u = 1;
% rr_tgt_ang_k = -60*pi/180;          



end

function end_effector = forward_kinematics(s, u, k, body)
% from center of the shoulder, 
l1 = body.upper_length;
l2 = body.lower_length;
end_effector = [ - l2*sin(k + u) - l1*sin(u);
  sin(s)*(l2*cos(k + u) + l1*cos(u));
 -cos(s)*(l2*cos(k + u) + l1*cos(u))  ]  ;

end

function [inv_s,inv_u,inv_k] = inverse_kinematics(p, body)
% from center of the shoulder
x = p(1);
y = p(2);
z = p(3);
l1 = body.upper_length;
l2 = body.lower_length;

inv_s = asin(y/sqrt(y*y+z*z));
inv_k = -acos((x*x+y*y+z*z-l1*l1-l2*l2)/(2*l1*l2)); % always assume knee is minus

if abs(inv_k) > 1e-4
    if abs(inv_s) > 1e-4
        temp1 = y/sin(inv_s)+(l2*cos(inv_k)+l1)*x/l2/sin(inv_k);
    else
        temp1 = -z/cos(inv_s)+(l2*cos(inv_k)+l1)*x/l2/sin(inv_k);
    end
    temp2 = -l2*sin(inv_k)-(l2*cos(inv_k)+l1)*(l2*cos(inv_k)+l1)/(l2*sin(inv_k));
    inv_u = asin(temp1/temp2);
else
    inv_u = asin(x/(-l1-l2));
end

end
